simulink model "SMC_equiv"  (R2024b)
settings: Solver=ode4  StartTime=0.0  StopTime=20  FixedStep=0.001  RelTol=1e-3
undefined symbols (not defined in the file or in its folder): a_smc_equiv, alpha_mrac, alpha_smc, beta_eq_smc, gamma_mrac, gamma_smc, gm_smc, theta_ref_smc
settings Model: Creator=juanm  LastModifiedBy=juanm

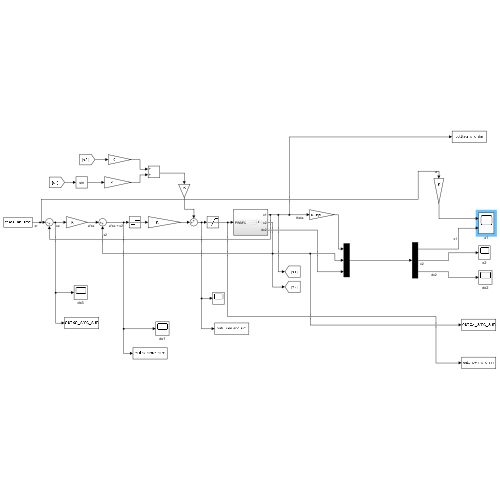
[thumbnail: Simulink's stored preview of the top-level diagram]
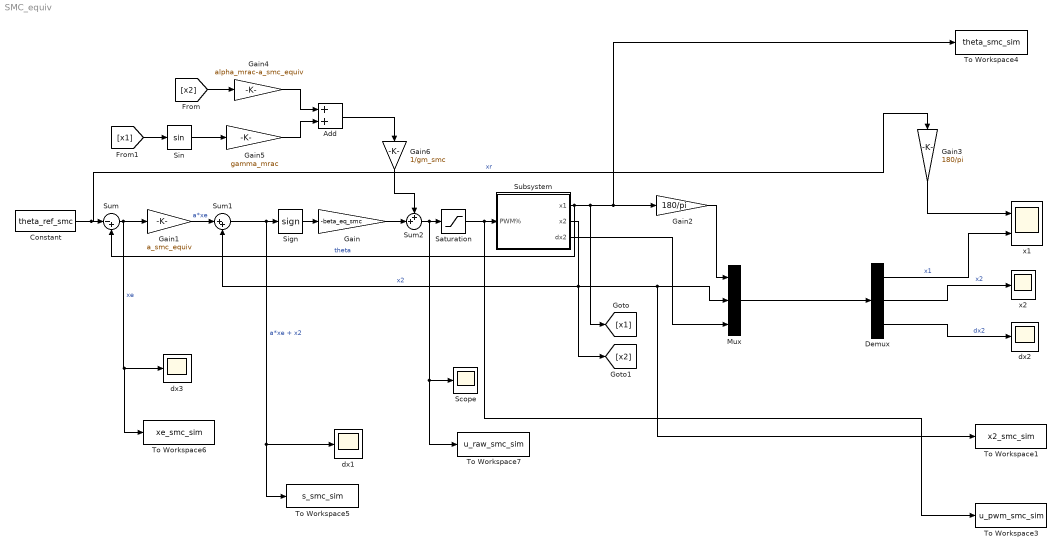
== system SMC_equiv ==
  Add : Sum
  Constant : Constant  Value=theta_ref_smc
  Demux : Demux  Outputs=3
  Gain : Gain  Gain=-beta_eq_smc
  Gain1 : Gain  Gain=a_smc_equiv
  Gain2 : Gain  Gain=180/pi
  Gain3 : Gain  Gain=180/pi
  Gain4 : Gain  Gain=alpha_mrac-a_smc_equiv
  Gain5 : Gain  Gain=gamma_mrac
  Gain6 : Gain  Gain=1/gm_smc
  Mux : Mux  Inputs=3
  Saturation : Saturate  UpperLimit=100  LowerLimit=0  ZeroCross=off
  Scope : Scope
  Sign : Signum  ZeroCross=off
  Sin : Trigonometry
  Subsystem : Subsystem
  Sum : Sum  Inputs=|-+
  Sum1 : Sum  Inputs=|++
  Sum2 : Sum  Inputs=++|
  To Workspace1 : ToWorkspace  VariableName=x2_smc_sim  SaveFormat=Timeseries  SampleTime=-1
  To Workspace3 : ToWorkspace  VariableName=u_pwm_smc_sim  SaveFormat=Timeseries  SampleTime=-1
  To Workspace4 : ToWorkspace  VariableName=theta_smc_sim  SaveFormat=Timeseries  SampleTime=-1
  To Workspace5 : ToWorkspace  VariableName=s_smc_sim  SaveFormat=Timeseries  SampleTime=-1
  To Workspace6 : ToWorkspace  VariableName=xe_smc_sim  SaveFormat=Timeseries  SampleTime=-1
  To Workspace7 : ToWorkspace  VariableName=u_raw_smc_sim  SaveFormat=Timeseries  SampleTime=-1
  dx1 : Scope
  dx2 : Scope
  dx3 : Scope
  x1 : Scope  NumInputPorts=2
  x2 : Scope
  wires:
  Sign/1 -> Gain/1
  Mux/1 -> Demux/1
  Demux/3 -> dx2/1  "dx2"
  Subsystem/2(x2) -> [x2], To Workspace1/1, Mux/2, Sum1/2  "x2"
  Constant/1 -> Gain3/1, Sum/1  "xr"
  Demux/1 -> x1/2  "x1"
  Gain1/1 -> Sum1/1  "a*xe"
  Sum/1 -> To Workspace6/1, dx3/1, Gain1/1  "xe"
  Sum1/1 -> dx1/1, To Workspace5/1, Sign/1  "a*xe + x2"
  Demux/2 -> x2/1  "x2"
  Subsystem/3(dx2) -> Mux/3
  Subsystem/1(x1) -> [x1], To Workspace4/1, Gain2/1, Sum/2  "theta"
  Saturation/1 -> To Workspace3/1, Subsystem/1(PWM%)
  Gain/1 -> Sum2/2
  Gain2/1 -> Mux/1
  Gain3/1 -> x1/1
  Sin/1 -> Gain5/1
  Gain4/1 -> Add/1
  Gain5/1 -> Add/2
  Add/1 -> Gain6/1
  [x2] -> Gain4/1
  [x1] -> Sin/1
  Sum2/1 -> Scope/1, To Workspace7/1, Saturation/1
  Gain6/1 -> Sum2/1

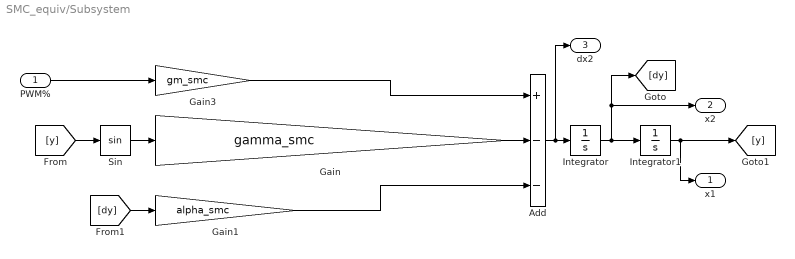
== system SMC_equiv/Subsystem ==
  PWM% : Inport
  Add : Sum  Inputs=+--
  Gain : Gain  Gain=gamma_smc
  Gain1 : Gain  Gain=alpha_smc
  Gain3 : Gain  Gain=gm_smc
  Integrator : Integrator
  Integrator1 : Integrator
  Sin : Trigonometry
  x1 : Outport
  x2 : Outport  Port=2
  dx2 : Outport  Port=3
  wires:
  Integrator/1 -> [dy], x2/1, Integrator1/1
  [dy] -> Gain1/1
  Add/1 -> dx2/1, Integrator/1
  Sin/1 -> Gain/1
  Gain/1 -> Add/2
  [y] -> Sin/1
  Gain1/1 -> Add/3
  PWM%/1 -> Gain3/1
  Gain3/1 -> Add/1
  Integrator1/1 -> [y], x1/1
